simulink model "HevP2TransmissionController"  (R2022a)
settings: Solver=FixedStepDiscrete  StartTime=0.0  StopTime=inf  FixedStep=0.01  RelTol=1e-3  EnableMultiTasking=on
model workspace (MAT data in the model file):
  Dn_Shft_Spd = Simulink.Parameter
  Dn_Shft_Spd.Value = [10.8  25.2  39.6  54  68.4; 10.8  25.2  39.6  54  68.4; 36  61.2  93.6  126  176.4; 36  61.2  93.6  126  176.4]
  Dn_Shft_Spd.DataType = 'double'
  Dn_Shft_Spd.Complexity = 'real'
  Dn_Shft_Spd.Dimensions = [4 5]
  Pdl_Pos_Dn_bpt = Simulink.Parameter
  Pdl_Pos_Dn_bpt.Value = [0 0.6 0.9 1]
  Pdl_Pos_Dn_bpt.DataType = 'double'
  Pdl_Pos_Dn_bpt.Complexity = 'real'
  Pdl_Pos_Dn_bpt.Dimensions = [1 4]
  Pdl_Pos_Up_bpt = Simulink.Parameter
  Pdl_Pos_Up_bpt.Value = [0 0.25 0.9 1]
  Pdl_Pos_Up_bpt.DataType = 'double'
  Pdl_Pos_Up_bpt.Complexity = 'real'
  Pdl_Pos_Up_bpt.Dimensions = [1 4]
  Up_Shft_Spd = Simulink.Parameter
  Up_Shft_Spd.Value = [18  32.4  46.8  61.2  75.6; 18  32.4  46.8  61.2  75.6; 43.2  68.4  100.8  133.2  183.6; 43.2  68.4  100.8  133.2  183.6]
  Up_Shft_Spd.DataType = 'double'
  Up_Shft_Spd.Complexity = 'real'
  Up_Shft_Spd.Dimensions = [4 5]
libraries: autolibtranscontrolscommon x1
settings Model: DataDictionary=HevP2TransmissionController.sldd  ModifiedByFormat=The MathWorks, Inc.  Creator=The MathWorks, Inc.  LastModifiedBy=The MathWorks, Inc.
settings SolverCC: AlgebraicLoopSolver=TrustRegion  AutoInsertRateTranBlk=on  MaxZcPerStep=1
settings DataIOCC: SaveOutput=off  SaveTime=off  ReturnWorkspaceOutputs=off
settings DebuggingCC: UnconnectedInputMsg=warning  UnconnectedOutputMsg=warning  UnconnectedLineMsg=warning  SFMachineParentedDataDiag=warning  ArithmeticOperatorsInVariantConditions=warning
settings SFSimCC: SimUseLocalCustomCode=off  CustomCodeUndefinedFunction=UseInterfaceOnly
settings RTWCC: RTWUseLocalCustomCode=off  DLArmComputeVersion=19.05
settings CodeAppCC: StateflowObjectComments=on

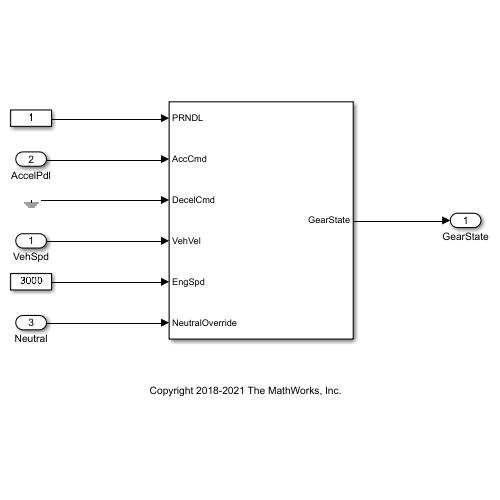
[thumbnail: Simulink's stored preview of the top-level diagram]
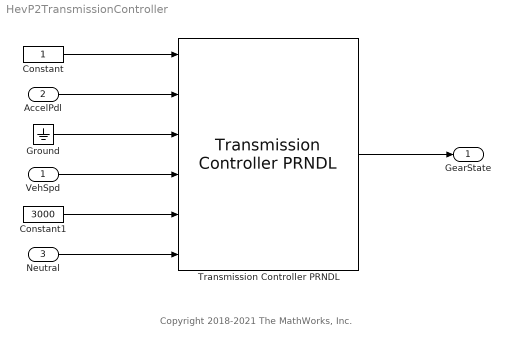
== system HevP2TransmissionController ==
  note: Copyright 2018-2021 The MathWorks, Inc.
  VehSpd : Inport  OutDataTypeStr=double  Unit=m/s  PortDimensions=1
  AccelPdl : Inport  Port=2  OutDataTypeStr=double  PortDimensions=1
  Neutral : Inport  Port=3
  Constant : Constant
  Constant1 : Constant  Value=3000
  Ground : Ground
  Transmission Controller PRNDL : autolibtranscontrolscommon/Transmission Controller PRNDL  GearInit=1  LugSpd=1200  MinUpSpd=1000  tClutchUp=0.5  tClutchDn=0.5  tPark=120  VelUnit=km/hr  UpShSpd=Up_Shft_Spd  UpLdBpt=Pdl_Pos_Up_bpt  UpShBpt=1:5  DnShSpd=Dn_Shft_Spd  DnLdBpt=Pdl_Pos_Dn_bpt  DnShBpt=2:6  POFS=zeros(4,1)  GOFS=zeros(1,5)  Ngears=6  aMode=1
      settings: SourceProductBaseCode=PW,DR,MT,VE
  GearState : Outport  VectorParamsAs1DForOutWhenUnconnected=off
  wires:
  Neutral/1 -> Transmission Controller PRNDL/6
  VehSpd/1 -> Transmission Controller PRNDL/4
  AccelPdl/1 -> Transmission Controller PRNDL/2
  Transmission Controller PRNDL/1 -> GearState/1
  Constant/1 -> Transmission Controller PRNDL/1
  Constant1/1 -> Transmission Controller PRNDL/5
  Ground/1 -> Transmission Controller PRNDL/3
